simulink library "dummySpool_cl"  (R2020a)
settings: Solver=VariableStepAuto  StartTime=0.0  StopTime=10.0  RelTol=1e-3
undefined symbols (not defined in the file or in its folder): a, courseFollow, courseFollow_cl, desiredMoment, env, exit, FLIGHTCONTROLLER, fltCtrl, freqRollYaw, initializeBussesFromBlock, pathFollowingController, pathFollowingController_cl, rollAmp, rollCtrlKd, rollCtrlKp, rollPhase, rollYawPeriod, takeOffToLandingExp, tsSpool, vhcl, xcurrent, yawAmp, yawCtrlKd, yawCtrlKp, yawPhase
libraries: simulink x4, filteredPIDController_ul x4, angleBtw2Vecs_ul x4, dspsigops x3, pathGeometry_ul x3, ctrlAllocMatrix3Comp_cl x2, setpointToOutput_cl x2, tanFrameProjection_ul x2, vectorNormalizer_ul x2, velocityAngle_ul x2, findClosestPointOnPath_new x1, eulAng2RotMat_ul x1
(part 1 of 2)
settings Model: Creator=jldanie5  LastModifiedBy=andre
settings DataIOCC: ReturnWorkspaceOutputs=off
settings DebuggingCC: ArithmeticOperatorsInVariantConditions=warning
settings SFSimCC: CustomCodeUndefinedFunction=UseInterfaceOnly

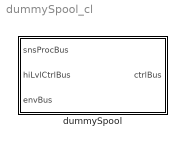
== system dummySpool_cl ==
  dummySpool : Subsystem  LoadFcn=initializeBussesFromBlock(gcb)  InitFcn=initializeBussesFromBlock(gcb)  StartFcn=initializeBussesFromBlock(gcb)  VariantControl=strcmpi(FLIGHTCONTROLLER,'takeoffToLanding')  mask{initPosForInitSStar=vhcl.initPosVecGnd.Value, fluidDensity=env.water.density.Value, pathCtrl=fltCtrl, aeroStruct=vhcl.struct('OCT.aeroSurf')}
      mask prompts: initPosForInitSStar "Initial Position"; fluidDensity "Fluid Density"; pathCtrl "Controller"; aeroStruct "Aerodynamic Structure"
      settings: MinAlgLoopOccurrences=on
      mask DialogControl Container3 Prompt: courseFollow Params
      mask DialogControl Container4 Prompt: setpointToOutput Params

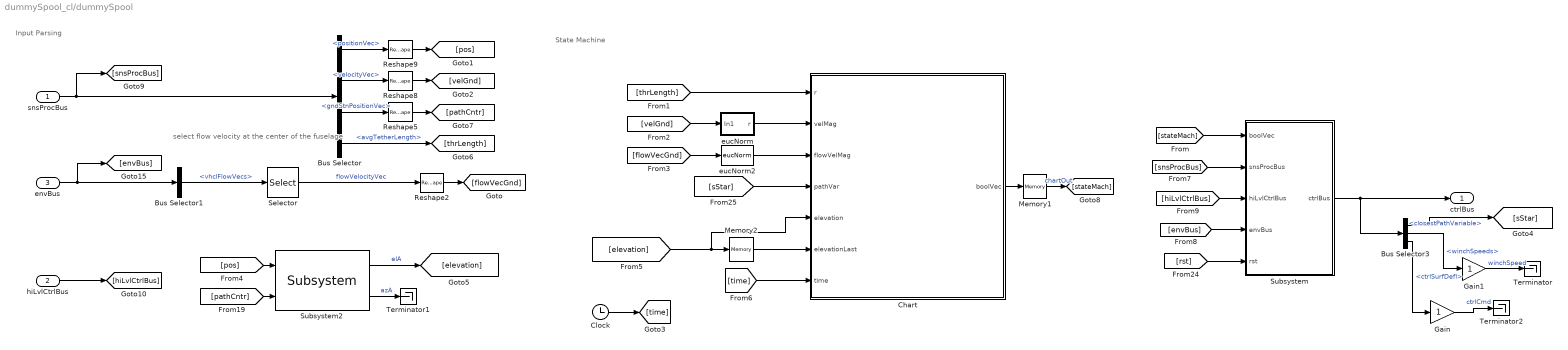
== system dummySpool_cl/dummySpool ==
  note: State Machine
  note: select flow velocity at the center of the fuselage
  note: Input Parsing
  snsProcBus : Inport  OutDataTypeStr=Bus: sensorsProcessingBus
  hiLvlCtrlBus : Inport  Port=2  OutDataTypeStr=Bus: hiLvlCtrlBus
  envBus : Inport  Port=3  OutDataTypeStr=Bus: envBus
  Bus Selector : BusSelector  OutputSignals=positionVec,velocityVec,gndStnPositionVec,avgTetherLength
  Bus Selector1 : BusSelector  OutputSignals=vhclFlowVecs
  Bus Selector3 : BusSelector  OutputSignals=closestPathVariable,winchSpeeds,ctrlSurfDefl
  Chart : Stateflow chart  TreatAsAtomicUnit=on  mask{gain41=fltCtrl.gain4to1.Value, gain23=fltCtrl.gain2to3.Value, maxR=fltCtrl.maxTL.Value, minTL=fltCtrl.initTL.Value, elvPeak=fltCtrl.elvPeak.Value}
      mask prompts: maxR "max kite position magnitude (r)"; minTL "minimum tether length"; elvPeak "elvation peak for phase 1"
  Clock : Clock
  Gain : Gain
  Gain1 : Gain
  Memory1 : Memory  InitialCondition=[1 0 0 0]
  Memory2 : Memory  InitialCondition=.36
  Reshape{2,5,8..9} (4 alike) : Reshape  OutputDimensionality=Column vector (2-D)
  Selector : Selector  NumberOfDimensions=2  InputPortWidth=3  IndexOptions=Select all,Index vector (dialog)  Indices=[1 3],5  OutputSizes=1,1
  Subsystem : Subsystem
  Subsystem2 : hiToLoElevationControllerExp/hiToLoElevationControllerExp/Subsystem  SystemSampleTime=-1  Latency=0  AutoFrameSizeCalculation=off
  Terminator : Terminator
  Terminator1 : Terminator
  Terminator2 : Terminator
  eucNorm : Subsystem
  eucNorm2 : takeoffToLanding_cl/takeoffToLanding/eucNorm  SystemSampleTime=-1  Latency=0  AutoFrameSizeCalculation=off
  ctrlBus : Outport  OutDataTypeStr=Bus: fltCtrlBus  VectorParamsAs1DForOutWhenUnconnected=off
  wires:
  snsProcBus/1 -> [snsProcBus], Bus Selector/1
  Bus Selector/2 -> Reshape8/1  "<velocityVec>"
  Bus Selector/1 -> Reshape9/1  "<positionVec>"
  Reshape2/1 -> [flowVecGnd]
  Reshape8/1 -> [velGnd]
  Reshape9/1 -> [pos]
  Selector/1 -> Reshape2/1  "flowVelocityVec"
  envBus/1 -> [envBus], Bus Selector1/1
  Bus Selector1/1 -> Selector/1  "<vhclFlowVecs>"
  Chart/1(boolVec) -> Memory1/1
  hiLvlCtrlBus/1 -> [hiLvlCtrlBus]
  [flowVecGnd] -> eucNorm2/1
  eucNorm/1(r) -> Chart/2(velMag)
  eucNorm2/1 -> Chart/3(flowVelMag)
  Memory1/1 -> [stateMach]  "chartOut"
  [elevation] -> Chart/5(elevation), Memory2/1
  Memory2/1 -> Chart/6(elevationLast)
  [time] -> Chart/7(time)
  Subsystem2/1 -> [elevation]  "elA"
  [pos] -> Subsystem2/1
  [pathCntr] -> Subsystem2/2
  Subsystem2/2 -> Terminator1/1  "azA"
  Reshape5/1 -> [pathCntr]
  Bus Selector/3 -> Reshape5/1  "<gndStnPositionVec>"
  [velGnd] -> eucNorm/1(In1)
  Bus Selector3/1 -> [sStar]  "<closestPathVariable>"
  [sStar] -> Chart/4(pathVar)
  Subsystem/1(ctrlBus) -> ctrlBus/1, Bus Selector3/1
  [snsProcBus] -> Subsystem/2(snsProcBus)
  [hiLvlCtrlBus] -> Subsystem/3(hiLvlCtrlBus)
  [envBus] -> Subsystem/4(envBus)
  [rst] -> Subsystem/5("rst ")
  [stateMach] -> Subsystem/1(boolVec)
  Bus Selector3/2 -> Gain1/1  "<winchSpeeds>"
  Clock/1 -> [time]
  Bus Selector3/3 -> Gain/1  "<ctrlSurfDefl>"
  Gain/1 -> Terminator2/1  "ctrlCmd"
  Gain1/1 -> Terminator/1  "winchSpeed"
  Bus Selector/4 -> [thrLength]  "<avgTetherLength>"
  [thrLength] -> Chart/1(r)

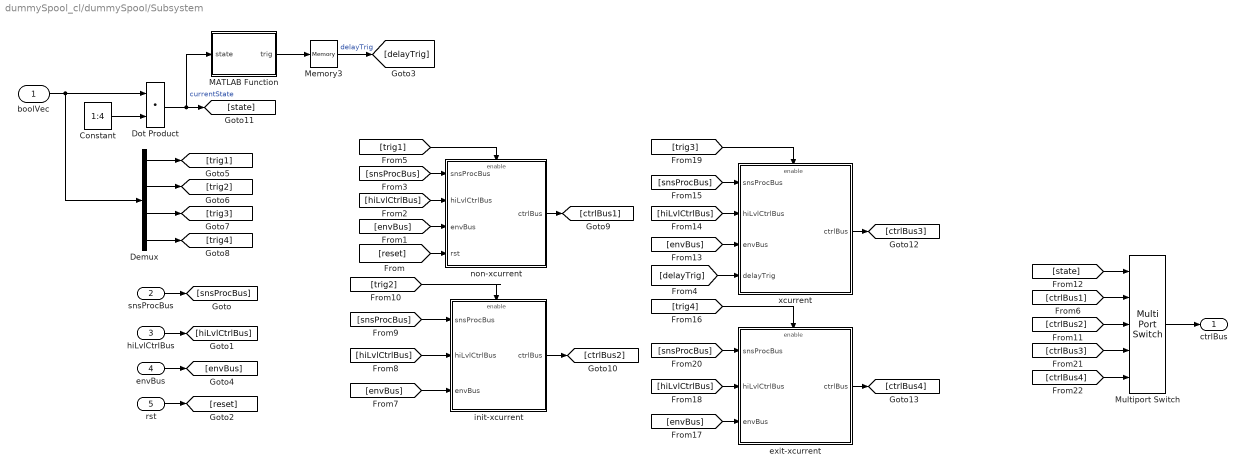
== system dummySpool_cl/dummySpool/Subsystem ==
  boolVec : Inport
  snsProcBus : Inport  Port=2
  hiLvlCtrlBus : Inport  Port=3
  envBus : Inport  Port=4
  "rst " : Inport  Port=5
  Constant : Constant  Value=1:4
  Demux : Demux
  Dot Product : DotProduct  InputSameDT=on  OutDataTypeStr=Inherit: Inherit via internal rule
  MATLAB Function : MATLAB Function  TreatAsAtomicUnit=on
  Memory3 : Memory
  Multiport Switch : MultiPortSwitch  Inputs=4  DataPortIndices={1,2,3,4,5,6}  DiagnosticForDefault=Warning
  exit-xcurrent : Subsystem  TreatAsAtomicUnit=on
  init-xcurrent : Subsystem  TreatAsAtomicUnit=on
  non-xcurrent : Subsystem  TreatAsAtomicUnit=on
  xcurrent : Subsystem  TreatAsAtomicUnit=on
  ctrlBus : Outport
  wires:
  [snsProcBus] -> init-xcurrent/1(snsProcBus)
  boolVec/1 -> Demux/1, Dot Product/1
  [hiLvlCtrlBus] -> init-xcurrent/2(hiLvlCtrlBus)
  Dot Product/1 -> [state], MATLAB Function/1(state)  "currentState"
  [envBus] -> init-xcurrent/3(envBus)
  Constant/1 -> Dot Product/2
  MATLAB Function/1(trig) -> Memory3/1
  Memory3/1 -> [delayTrig]  "delayTrig"
  Multiport Switch/1 -> ctrlBus/1
  [delayTrig] -> xcurrent/4(delayTrig)
  snsProcBus/1 -> [snsProcBus]
  envBus/1 -> [envBus]
  "rst "/1 -> [reset]
  hiLvlCtrlBus/1 -> [hiLvlCtrlBus]
  [reset] -> non-xcurrent/4("rst ")
  [envBus] -> non-xcurrent/3(envBus)
  [hiLvlCtrlBus] -> non-xcurrent/2(hiLvlCtrlBus)
  [snsProcBus] -> non-xcurrent/1(snsProcBus)
  Demux/1 -> [trig1]
  Demux/2 -> [trig2]
  Demux/3 -> [trig3]
  Demux/4 -> [trig4]
  [trig1] -> non-xcurrent/Enable
  non-xcurrent/1(ctrlBus) -> [ctrlBus1]
  [ctrlBus1] -> Multiport Switch/2
  [trig2] -> init-xcurrent/Enable
  init-xcurrent/1(ctrlBus) -> [ctrlBus2]
  [ctrlBus2] -> Multiport Switch/3
  [state] -> Multiport Switch/1
  [snsProcBus] -> xcurrent/1(snsProcBus)
  [hiLvlCtrlBus] -> xcurrent/2(hiLvlCtrlBus)
  [envBus] -> xcurrent/3(envBus)
  [trig3] -> xcurrent/Enable
  [trig4] -> exit-xcurrent/Enable
  [snsProcBus] -> exit-xcurrent/1(snsProcBus)
  [hiLvlCtrlBus] -> exit-xcurrent/2(hiLvlCtrlBus)
  [envBus] -> exit-xcurrent/3(envBus)
  xcurrent/1(ctrlBus) -> [ctrlBus3]
  exit-xcurrent/1(ctrlBus) -> [ctrlBus4]
  [ctrlBus3] -> Multiport Switch/4
  [ctrlBus4] -> Multiport Switch/5

== system dummySpool_cl/dummySpool/eucNorm ==
  In1 : Inport
  Dot Product1 : DotProduct  InputSameDT=on  OutDataTypeStr=Inherit: Inherit via internal rule
  Reshape1 : Reshape
  Sqrt : Sqrt  SaturateOnIntegerOverflow=on
  r : Outport
  wires:
  Sqrt/1 -> Reshape1/1
  In1/1 -> Dot Product1/2, Dot Product1/1
  Reshape1/1 -> r/1  "r"
  Dot Product1/1 -> Sqrt/1

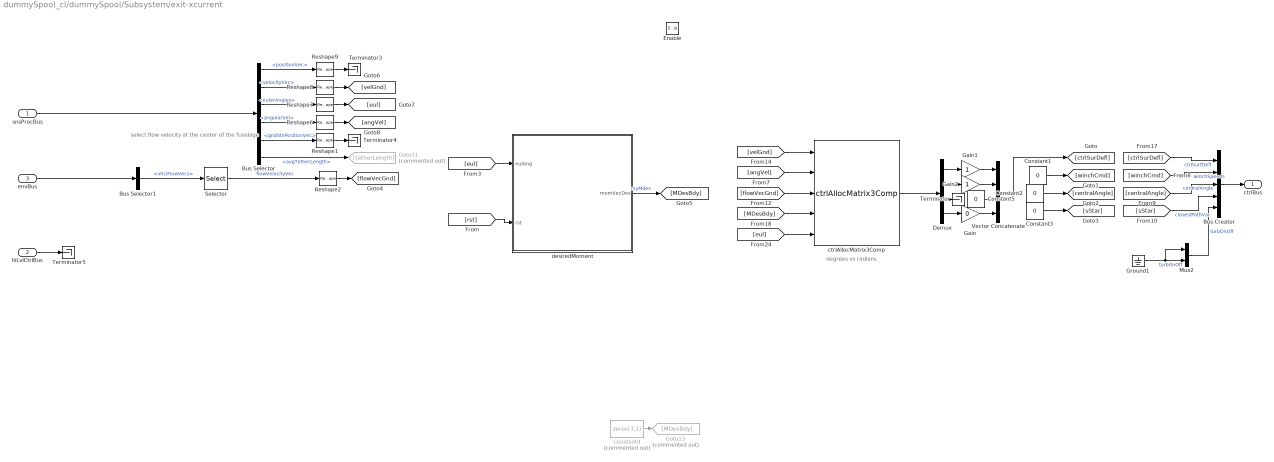
== system dummySpool_cl/dummySpool/Subsystem/exit-xcurrent ==
  note: degrees vs radians
  note: select flow velocity at the center of the fuselage
  snsProcBus : Inport  OutDataTypeStr=Bus: sensorsProcessingBus
  hiLvlCtrlBus : Inport  Port=2  OutDataTypeStr=Bus: hiLvlCtrlBus
  envBus : Inport  Port=3  OutDataTypeStr=Bus: envBus
  Enable : EnablePort
  Bus Creator : BusCreator  Inputs=5  OutDataTypeStr=Bus: fltCtrlBus
      settings: InheritFromInputs=off
  Bus Selector : BusSelector  OutputSignals=positionVec,velocityVec,eulerAngles,angularVel,gndStnPositionVec,avgTetherLength
  Bus Selector1 : BusSelector  OutputSignals=vhclFlowVecs
  Constant{1..3,5} (4 alike) : Constant  Value=0
  Constant4 : Constant  Commented=on  Value=zeros(3,1)
  Demux : Demux
  Gain : Gain  Gain=0
  Gain1 : Gain
  Gain2 : Gain
  Goto11 : Goto  Commented=on  GotoTag=tetherLength
  Goto13 : Goto  Commented=on  GotoTag=MDesBdy
  Ground1 : Ground
  Mux2 : Mux  Inputs=2
  Reshape{1..2,6..9} (6 alike) : Reshape  OutputDimensionality=Column vector (2-D)
  Selector : Selector  NumberOfDimensions=2  InputPortWidth=3  IndexOptions=Select all,Index vector (dialog)  Indices=[1 3],5  OutputSizes=1,1
  Terminator{,3..5} (4 alike) : Terminator
  Vector Concatenate : Concatenate  NumInputs=4
  ctrlAllocMatrix3Comp : ctrlAllocMatrix3Comp_cl/ctrlAllocMatrix3Comp  aeroStruct=vhcl.struct('OCT.aeroSurf')  fluidDensity=fluidDensity  arms=vhcl.struct('OCT.thrAttch')
  desiredMoment : Subsystem  AncestorBlock=takeOffToLandingExp/takeOffToLandingExp/exit-xcurrent/desiredMoment
  ctrlBus : Outport  OutDataTypeStr=Bus: fltCtrlBus  VectorParamsAs1DForOutWhenUnconnected=off
  wires:
  [sStar] -> Bus Creator/4  "closestPathVar"
  [ctrlSurDefl] -> Bus Creator/1  "ctrlSurfDefl"
  [winchCmd] -> Bus Creator/2  "winchSpeeds"
  Bus Creator/1 -> ctrlBus/1
  [centralAngle] -> Bus Creator/3  "centralAngle"
  Constant1/1 -> [winchCmd]
  Constant2/1 -> [centralAngle]
  Constant3/1 -> [sStar]
  Bus Selector/1 -> Reshape9/1  "<positionVec>"
  Bus Selector/3 -> Reshape7/1  "<eulerAngles>"
  Bus Selector/2 -> Reshape8/1  "<velocityVec>"
  Reshape7/1 -> [eul]
  Bus Selector/4 -> Reshape6/1  "<angularVel>"
  Reshape8/1 -> [velGnd]
  Selector/1 -> Reshape2/1  "flowVelocityVec"
  Reshape9/1 -> Terminator3/1
  Bus Selector/5 -> Reshape1/1  "<gndStnPositionVec>"
  Reshape2/1 -> [flowVecGnd]
  Bus Selector1/1 -> Selector/1  "<vhclFlowVecs>"
  envBus/1 -> Bus Selector1/1
  Reshape1/1 -> Terminator4/1
  snsProcBus/1 -> Bus Selector/1
  Reshape6/1 -> [angVel]
  [flowVecGnd] -> ctrlAllocMatrix3Comp/3
  [angVel] -> ctrlAllocMatrix3Comp/2
  [eul] -> ctrlAllocMatrix3Comp/5
  [MDesBdy] -> ctrlAllocMatrix3Comp/4
  [velGnd] -> ctrlAllocMatrix3Comp/1
  Bus Selector/6 -> Goto11/1  "<avgTetherLength>"
  ctrlAllocMatrix3Comp/1 -> Demux/1
  Vector Concatenate/1 -> [ctrlSurDefl]
  Demux/1 -> Gain1/1
  Demux/2 -> Gain2/1
  Demux/4 -> Gain/1
  Constant4/1 -> Goto13/1
  hiLvlCtrlBus/1 -> Terminator5/1
  Constant5/1 -> Vector Concatenate/3
  Demux/3 -> Terminator/1
  desiredMoment/1(momVecDes) -> [MDesBdy]  "myMdes"
  [eul] -> desiredMoment/1(eulAng)
  [rst] -> desiredMoment/2(rst)
  Gain/1 -> Vector Concatenate/4
  Gain1/1 -> Vector Concatenate/1
  Gain2/1 -> Vector Concatenate/2
  Mux2/1 -> Bus Creator/5  "turbOnOff"
  Ground1/1 -> Mux2/2, Mux2/1  "turbOnOff"

== system dummySpool_cl/dummySpool/Subsystem/init-xcurrent ==
  snsProcBus : Inport  OutDataTypeStr=Bus: sensorsProcessingBus
  hiLvlCtrlBus : Inport  Port=2  OutDataTypeStr=Bus: hiLvlCtrlBus
  envBus : Inport  Port=3  OutDataTypeStr=Bus: envBus
  Enable : EnablePort
  Bus Creator : BusCreator  Inputs=5  OutDataTypeStr=Bus: fltCtrlBus
      settings: InheritFromInputs=off
  Constant : Constant  Value=[0 0 fltCtrl.phase2Elevator.Value 0]'
  Constant1 : Constant  Value=0
  Constant2 : Constant  Value=0
  Constant3 : Constant  Value=0
  Ground{,1..3} (4 alike) : Ground
  Mux2 : Mux  Inputs=2
  Terminator : Terminator
  Terminator1 : Terminator
  Terminator2 : Terminator
  ctrlBus : Outport  OutDataTypeStr=Bus: fltCtrlBus  VectorParamsAs1DForOutWhenUnconnected=off
  wires:
  [ctrlSurDefl] -> Bus Creator/1  "ctrlSurfDefl"
  Ground1/1 -> Bus Creator/3  "centralAngle"
  Ground/1 -> Bus Creator/2  "winchSpeeds"
  envBus/1 -> Terminator1/1
  hiLvlCtrlBus/1 -> Terminator2/1
  Constant2/1 -> [centralAngle]
  snsProcBus/1 -> Terminator/1
  Ground2/1 -> Bus Creator/4  "closestPathVariable"
  Constant1/1 -> [winchCmd]
  Bus Creator/1 -> ctrlBus/1
  Constant3/1 -> [sStar]
  Constant/1 -> [ctrlSurDefl]
  Ground3/1 -> Mux2/2, Mux2/1  "turbOnOff"
  Mux2/1 -> Bus Creator/5  "turbOnOff"

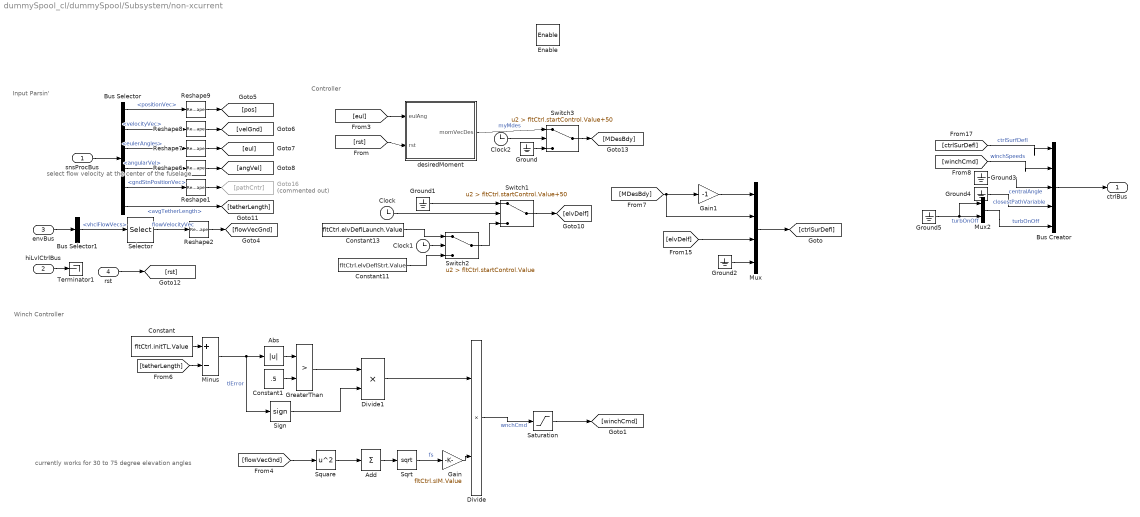
== system dummySpool_cl/dummySpool/Subsystem/non-xcurrent ==
  note: Controller
  note: Input Parsin'
  note: Winch Controller
  note: select flow velocity at the center of the fuselage
  note: currently works for 30 to 75 degree elevation angles
  snsProcBus : Inport  OutDataTypeStr=Bus: sensorsProcessingBus
  hiLvlCtrlBus : Inport  Port=2  OutDataTypeStr=Bus: hiLvlCtrlBus
  envBus : Inport  Port=3  OutDataTypeStr=Bus: envBus
  "rst " : Inport  Port=4
  Enable : EnablePort
  Abs : Abs
  Add : Sum  Inputs=+
  Bus Creator : BusCreator  Inputs=5  OutDataTypeStr=Bus: fltCtrlBus
      settings: InheritFromInputs=off
  Bus Selector : BusSelector  OutputSignals=positionVec,velocityVec,eulerAngles,angularVel,gndStnPositionVec,avgTetherLength
  Bus Selector1 : BusSelector  OutputSignals=vhclFlowVecs
  Clock : Clock
  Clock1 : Clock
  Clock2 : Clock
  Constant : Constant  Value=fltCtrl.initTL.Value
  Constant1 : Constant  Value=.5
  Constant11 : Constant  Value=fltCtrl.elvDeflStrt.Value
  Constant13 : Constant  Value=fltCtrl.elvDeflLaunch.Value
  Divide : Product  Inputs=**
  Divide1 : Product  Inputs=**
  Gain : Gain  Gain=fltCtrl.sIM.Value
  Gain1 : Gain  Gain=-1
  Goto16 : Goto  Commented=on  GotoTag=pathCntr
  GreaterThan : RelationalOperator  Operator=>  OutDataTypeStr=boolean  RndMeth=Simplest
  Ground{,1..5} (6 alike) : Ground
  Minus : Sum  Inputs=+-
  Mux : Mux
  Mux2 : Mux  Inputs=2
  Reshape{1..2,6..9} (6 alike) : Reshape  OutputDimensionality=Column vector (2-D)
  Saturation : Saturate  UpperLimit=0  LowerLimit=-inf
  Selector : Selector  NumberOfDimensions=2  InputPortWidth=3  IndexOptions=Select all,Index vector (dialog)  Indices=[1 3],5  OutputSizes=1,1
  Sign : Signum
  Sqrt : Sqrt  SaturateOnIntegerOverflow=on
  Square : Math  Operator=square  SignedPower=on  SaturateOnIntegerOverflow=on
  Switch1 : Switch  Criteria=u2 > Threshold  Threshold=fltCtrl.startControl.Value+50
  Switch2 : Switch  Criteria=u2 > Threshold  Threshold=fltCtrl.startControl.Value
  Switch3 : Switch  Criteria=u2 > Threshold  Threshold=fltCtrl.startControl.Value+50
  Terminator1 : Terminator
  desiredMoment : Subsystem
  ctrlBus : Outport  OutDataTypeStr=Bus: fltCtrlBus  VectorParamsAs1DForOutWhenUnconnected=off
  wires:
  Ground4/1 -> Bus Creator/4  "closestPathVariable"
  [ctrlSurDefl] -> Bus Creator/1  "ctrlSurfDefl"
  [winchCmd] -> Bus Creator/2  "winchSpeeds"
  Bus Creator/1 -> ctrlBus/1
  Ground3/1 -> Bus Creator/3  "centralAngle"
  desiredMoment/1(momVecDes) -> Switch3/1  "myMdes"
  Bus Selector/1 -> Reshape9/1  "<positionVec>"
  Bus Selector/3 -> Reshape7/1  "<eulerAngles>"
  Bus Selector/2 -> Reshape8/1  "<velocityVec>"
  Reshape7/1 -> [eul]
  Bus Selector/4 -> Reshape6/1  "<angularVel>"
  Reshape8/1 -> [velGnd]
  Selector/1 -> Reshape2/1  "flowVelocityVec"
  Reshape9/1 -> [pos]
  Bus Selector/5 -> Reshape1/1  "<gndStnPositionVec>"
  Reshape2/1 -> [flowVecGnd]
  Bus Selector1/1 -> Selector/1  "<vhclFlowVecs>"
  envBus/1 -> Bus Selector1/1
  Reshape1/1 -> Goto16/1
  snsProcBus/1 -> Bus Selector/1
  Reshape6/1 -> [angVel]
  [eul] -> desiredMoment/1(eulAng)
  [flowVecGnd] -> Square/1
  Add/1 -> Sqrt/1
  Bus Selector/6 -> [tetherLength]  "<avgTetherLength>"
  Constant/1 -> Minus/1
  Minus/1 -> Sign/1, Abs/1  "tlError"
  [tetherLength] -> Minus/2
  Sqrt/1 -> Gain/1  "fs"
  Square/1 -> Add/1
  "rst "/1 -> [rst]
  hiLvlCtrlBus/1 -> Terminator1/1
  [rst] -> desiredMoment/2(rst)
  Mux/1 -> [ctrlSurDefl]
  Abs/1 -> GreaterThan/1
  Constant1/1 -> GreaterThan/2
  Gain/1 -> Divide/2
  Divide/1 -> Saturation/1  "wnchCmd"
  Sign/1 -> Divide1/2
  Divide1/1 -> Divide/1
  GreaterThan/1 -> Divide1/1
  Saturation/1 -> [winchCmd]
  [elvDelf] -> Mux/3
  Constant11/1 -> Switch2/3
  Clock/1 -> Switch1/2
  Ground2/1 -> Mux/4
  Switch1/1 -> [elvDelf]
  Switch2/1 -> Switch1/3
  Clock1/1 -> Switch2/2
  Constant13/1 -> Switch2/1
  Switch3/1 -> [MDesBdy]
  Clock2/1 -> Switch3/2
  Gain1/1 -> Mux/1
  [MDesBdy] -> Mux/2, Gain1/1
  Ground/1 -> Switch3/3
  Ground1/1 -> Switch1/1
  Mux2/1 -> Bus Creator/5  "turbOnOff"
  Ground5/1 -> Mux2/2, Mux2/1  "turbOnOff"

== system dummySpool_cl/dummySpool/Subsystem/xcurrent ==
  snsProcBus : Inport  OutDataTypeStr=Bus: sensorsProcessingBus
  hiLvlCtrlBus : Inport  Port=2  OutDataTypeStr=Bus: hiLvlCtrlBus
  envBus : Inport  Port=3  OutDataTypeStr=Bus: envBus
  delayTrig : Inport  Port=4
  Enable : EnablePort
  Constant : Constant  Value=fltCtrl.controllerEnable.Value
  Switch : Switch  Criteria=u2 > Threshold
  pathFollowingController : Subsystem  Commented=on  AncestorBlock=pathFollowingController_cl/pathFollowingController  LoadFcn=initializeBussesFromBlock(gcb)  InitFcn=initializeBussesFromBlock(gcb)  StartFcn=initializeBussesFromBlock(gcb)  VariantControl=strcmpi(FLIGHTCONTROLLER,'pathFollowingController')  mask{initPosForInitSStar=vhcl.initPosVecGnd.Value, fluidDensity=env.water.density.Value, pathCtrl=fltCtrl, aeroStruct=vhcl.struct('OCT.aeroSurf')}
      mask prompts: initPosForInitSStar "Initial Position"; fluidDensity "Fluid Density"; pathCtrl "Controller"; aeroStruct "Aerodynamic Structure"
      settings: MinAlgLoopOccurrences=on
      mask DialogControl Container3 Prompt: courseFollow Params
      mask DialogControl Container4 Prompt: setpointToOutput Params
  pathFollowingControllerExpStateMachine : pathFollowingControllerExpStateMachine_cl/pathFollowingControllerExpStateMachine  VariantControl=strcmpi(FLIGHTCONTROLLER,'pathFollowingControllerMantaBandLin')  initPosForInitSStar=vhcl.initPosVecGnd.Value  fluidDensity=env.water.density.Value  pathCtrl=fltCtrl  aeroStruct=vhcl.struct('OCT.aeroSurf')  thrAttach=vhcl.rBridle_LE.Value  vhcl=vhcl
  periodicCtrlExpStateMachine : periodicCtrlExpStateMachine/periodicCtrlExpStateMachine  fltCtrl=fltCtrl
  ctrlBus : Outport  OutDataTypeStr=Bus: fltCtrlBus  VectorParamsAs1DForOutWhenUnconnected=off
  wires:
  delayTrig/1 -> [delayTrig]
  [snsProcBus] -> pathFollowingControllerExpStateMachine/1
  [hiLvlCtrlBus] -> pathFollowingControllerExpStateMachine/2
  [envBus] -> pathFollowingControllerExpStateMachine/3
  envBus/1 -> [envBus]
  hiLvlCtrlBus/1 -> [hiLvlCtrlBus]
  snsProcBus/1 -> [snsProcBus]
  [envBus] -> periodicCtrlExpStateMachine/3
  [hiLvlCtrlBus] -> periodicCtrlExpStateMachine/2
  [snsProcBus] -> periodicCtrlExpStateMachine/1
  Switch/1 -> ctrlBus/1
  pathFollowingControllerExpStateMachine/1 -> Switch/1
  periodicCtrlExpStateMachine/1 -> Switch/3
  Constant/1 -> Switch/2
  [delayTrig] -> periodicCtrlExpStateMachine/4
  [delayTrig] -> pathFollowingControllerExpStateMachine/4

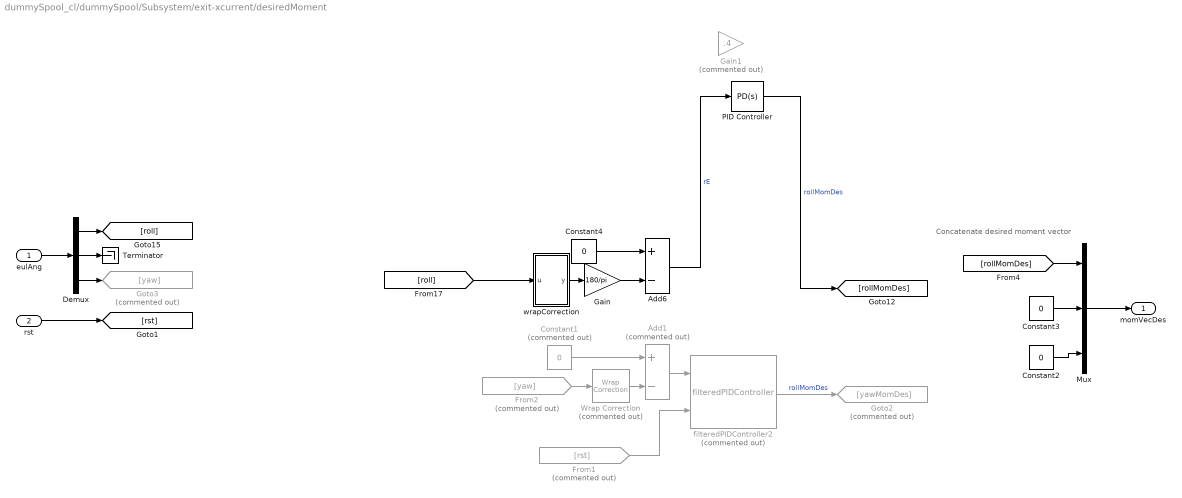
== system dummySpool_cl/dummySpool/Subsystem/exit-xcurrent/desiredMoment ==
  note: Concatenate desired moment vector
  eulAng : Inport
  rst : Inport  Port=2
  Add1 : Sum  Commented=on  Inputs=+-
  Add6 : Sum  Inputs=+-
  Constant1 : Constant  Commented=on  Value=0
  Constant2 : Constant  Value=0
  Constant3 : Constant  Value=0
  Constant4 : Constant  Value=0
  Demux : Demux  Outputs=3
  From1 : From  Commented=on  GotoTag=rst
  From2 : From  Commented=on  GotoTag=yaw
  Gain : Gain  Gain=180/pi
  Gain1 : Gain  Commented=on  Gain=.4
  Goto2 : Goto  Commented=on  GotoTag=yawMomDes
  Goto3 : Goto  Commented=on  GotoTag=yaw
  Mux : Mux  Inputs=3
  PID Controller : simulink/Continuous/PID Controller  Controller=PD  Form=Parallel  TimeDomain=Continuous-time  UseExternalTs=off  SampleTime=-1  IntegratorMethod=Forward Euler  FilterMethod=Forward Euler  ControllerParametersSource=internal  P=fltCtrl.rollMomentPhase1.kp.Value  I=1  D=fltCtrl.rollMomentPhase1.kd.Value  UseFilter=on  N=fltCtrl.rollMomentPhase1.tau.Value  TunerSelectOption=Transfer Function Based (PID Tuner App)  InitialConditionSource=internal  InitialConditionForIntegrator=0  InitialConditionForFilter=0  DifferentiatorICPrevScaledInput=0  ExternalReset=none  TrackingMode=off  Kt=1  LimitOutput=off  UpperSaturationLimit=inf  LowerSaturationLimit=-inf  LinearizeAsGain=on  AntiWindupMode=none  Kb=1  POutMin=[]  POutMax=[]  IOutMin=[]  IOutMax=[]  DOutMin=[]  DOutMax=[]  NOutMin=[]  NOutMax=[]  SumOutMin=[]  SumOutMax=[]  SaturationOutMin=[]  SaturationOutMax=[]  PParamMin=[]  PParamMax=[]  IParamMin=[]  IParamMax=[]  DParamMin=[]  DParamMax=[]  NParamMin=[]  NParamMax=[]  KbParamMin=[]  KbParamMax=[]  KtParamMin=[]  KtParamMax=[]  KbOutMin=[]  KbOutMax=[]  KtOutMin=[]  KtOutMax=[]  IntegratorOutMin=[]  IntegratorOutMax=[]  FilterOutMin=[]  FilterOutMax=[]  SumI1OutMin=[]  SumI1OutMax=[]  SumI2OutMin=[]  SumI2OutMax=[]  SumI3OutMin=[]  SumI3OutMax=[]  SumI4OutMin=[]  SumI4OutMax=[]  SumDOutMin=[]  SumDOutMax=[]  DifferentiatorOutMin=[]  DifferentiatorOutMax=[]  FilterDiffOutCoefMin=[]  FilterDiffOutCoefMax=[]  ReciprocalOutMin=[]  ReciprocalOutMax=[]  SumDenOutMin=[]  SumDenOutMax=[]  SumNumOutMin=[]  SumNumOutMax=[]  DivideOutMin=[]  DivideOutMax=[]  UdiffTsProdOutMin=[]  UdiffTsProdOutMax=[]  NTsProdOutMin=[]  NTsProdOutMax=[]  UintegralTsProdOutMin=[]  UintegralTsProdOutMax=[]  UngainTsProdOutMin=[]  UngainTsProdOutMax=[]  IntegratorContinuousStateAttributes=''  IntegratorStateMustResolveToSignalObject=off  IntegratorRTWStateStorageClass=Auto  FilterContinuousStateAttributes=''  FilterStateMustResolveToSignalObject=off  FilterRTWStateStorageClass=Auto  ParallelPVariant=InternalParameters  IdealPVariant=Disabled  IVariant=Disabled  DVariant=InternalParameters  IntegratorVariant=Disabled  SatVariant=Disabled  AWVariant=Disabled  PCopyVariant=Disabled  TRVariant=Disabled  FdbkBlocksVariant=Forward  IdealPFdbkVariant=Disabled  SatFdbkVariant=Disabled  DerivativeFilterVariant=ContFilter  NVariant=InternalParameters  NCopyVariant=Disabled  FilterICVariant=InternalICsFilter  IntegratorICVariant=Disabled  ExternalResetVariant=Disabled  TRSumVariant=Passthrough  SumFdbkVariant=Disabled  SumVariant=Sum_PD  TsampFilterVariant=InternalTs  TsampNgainVariant=Passthrough  TsampIntegralVariant=Disabled_SignalSpec
  Terminator : Terminator
  Wrap Correction : setpointToOutput_cl/desiredMoment/Wrap Correction  Commented=on  SystemSampleTime=-1  Latency=0  AutoFrameSizeCalculation=off
  filteredPIDController2 : filteredPIDController_ul/filteredPIDController  Commented=on  kp=pathCtrl.yawMoment.kp.Value  ki=0  kd=pathCtrl.yawMoment.kd.Value  Value=pathCtrl.yawMoment.tau.Value  externalReset=rising
  wrapCorrection : Subsystem
  momVecDes : Outport  VectorParamsAs1DForOutWhenUnconnected=off
  wires:
  Wrap Correction/1 -> Add1/2
  From2/1 -> Wrap Correction/1
  Constant1/1 -> Add1/1
  filteredPIDController2/1 -> Goto2/1  "rollMomDes"
  Add1/1 -> filteredPIDController2/1
  From1/1 -> filteredPIDController2/2
  rst/1 -> [rst]
  Demux/3 -> Goto3/1
  Demux/2 -> Terminator/1
  Constant4/1 -> Add6/1
  Add6/1 -> PID Controller/1  "rE"
  PID Controller/1 -> [rollMomDes]  "rollMomDes"
  eulAng/1 -> Demux/1
  Demux/1 -> [roll]
  Mux/1 -> momVecDes/1
  Constant3/1 -> Mux/2
  [rollMomDes] -> Mux/1
  Constant2/1 -> Mux/3
  Gain/1 -> Add6/2
  [roll] -> wrapCorrection/1(u)
  wrapCorrection/1(y) -> Gain/1

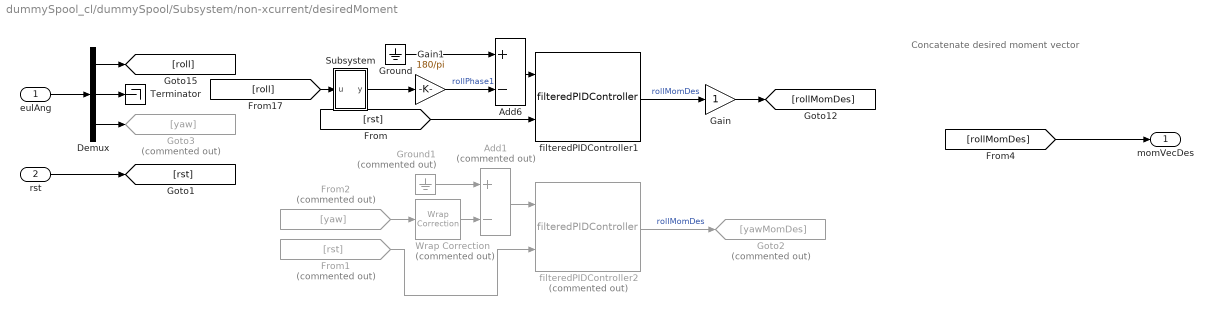
== system dummySpool_cl/dummySpool/Subsystem/non-xcurrent/desiredMoment ==
  note: Concatenate desired moment vector
  eulAng : Inport
  rst : Inport  Port=2
  Add1 : Sum  Commented=on  Inputs=+-
  Add6 : Sum  Inputs=+-
  Demux : Demux  Outputs=3
  From1 : From  Commented=on  GotoTag=rst
  From2 : From  Commented=on  GotoTag=yaw
  Gain : Gain
  Gain1 : Gain  Gain=180/pi
  Goto2 : Goto  Commented=on  GotoTag=yawMomDes
  Goto3 : Goto  Commented=on  GotoTag=yaw
  Ground : Ground
  Ground1 : Ground  Commented=on
  Subsystem : Subsystem
  Terminator : Terminator
  Wrap Correction : setpointToOutput_cl/desiredMoment/Wrap Correction  Commented=on  SystemSampleTime=-1  Latency=0  AutoFrameSizeCalculation=off
  filteredPIDController1 : filteredPIDController_ul/filteredPIDController  kp=fltCtrl.rollMomentPhase1.kp.Value  ki=0  kd=fltCtrl.rollMomentPhase1.kd.Value  Value=fltCtrl.rollMomentPhase1.tau.Value  externalReset=rising
  filteredPIDController2 : filteredPIDController_ul/filteredPIDController  Commented=on  kp=pathCtrl.yawMoment.kp.Value  ki=0  kd=pathCtrl.yawMoment.kd.Value  Value=pathCtrl.yawMoment.tau.Value  externalReset=rising
  momVecDes : Outport  VectorParamsAs1DForOutWhenUnconnected=off
  wires:
  Demux/1 -> [roll]
  eulAng/1 -> Demux/1
  filteredPIDController1/1 -> Gain/1  "rollMomDes"
  Add6/1 -> filteredPIDController1/1
  Demux/2 -> Terminator/1
  Demux/3 -> Goto3/1
  rst/1 -> [rst]
  [rst] -> filteredPIDController1/2
  From1/1 -> filteredPIDController2/2
  Add1/1 -> filteredPIDController2/1
  filteredPIDController2/1 -> Goto2/1  "rollMomDes"
  From2/1 -> Wrap Correction/1
  Wrap Correction/1 -> Add1/2
  Gain/1 -> [rollMomDes]
  Gain1/1 -> Add6/2  "rollPhase1"
  [rollMomDes] -> momVecDes/1
  Ground/1 -> Add6/1
  Ground1/1 -> Add1/1
  [roll] -> Subsystem/1(u)
  Subsystem/1(y) -> Gain1/1

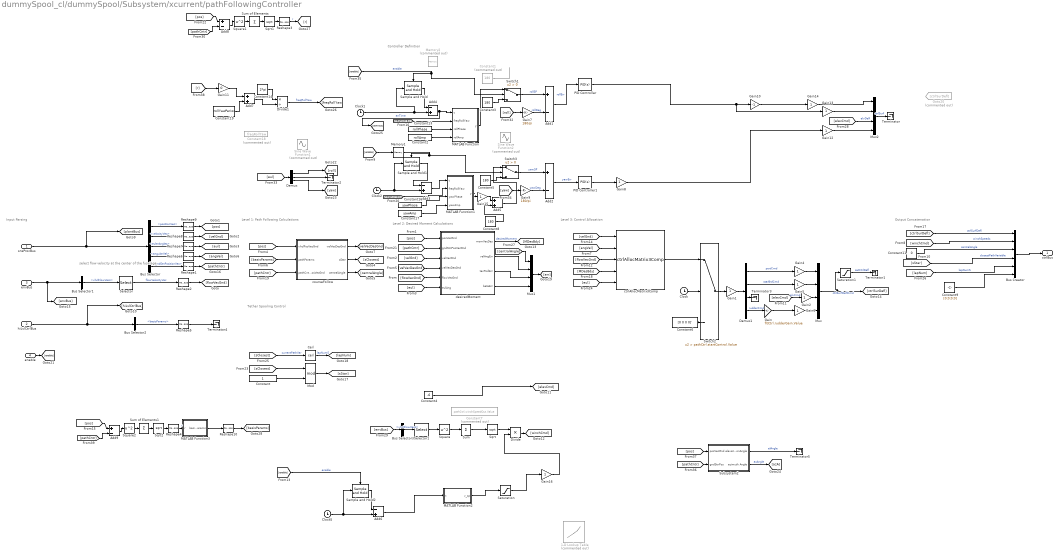
== system dummySpool_cl/dummySpool/Subsystem/xcurrent/pathFollowingController ==
  note: Input Parsing
  note: Level 1: Path Following Calculations
  note: Level 2: Desired Moment Calculations
  note: Tether Spooling Control
  note: Output Concatenation
  note: Level 3: Control Allocation
  note: select flow velocity at the center of the fuselage
  note: Controller Definition
  snsProcBus : Inport  OutDataTypeStr=Bus: sensorsProcessingBus
  hiLvlCtrlBus : Inport  Port=2  OutDataTypeStr=Bus: hiLvlCtrlBus
  envBus : Inport  Port=3  OutDataTypeStr=Bus: envBus
  enable : Inport  Port=4
  1-D Lookup Table : Lookup_n-D  Commented=on  NumberOfTableDimensions=1  BreakpointsForDimension1=tsSpool.Time  Table=tsSpool.Data  ExtrapMethod=Clip  InternalRulePriority=Speed  RndMeth=Simplest  InputSameDT=on
  Add{1..2,8..9} (4 alike) : Sum  Inputs=+-
  Add3 : Sum  Inputs=-+
  Add4 : Sum  Inputs=-+
  Add5 : Sum
  Add6 : Sum  Inputs=-+
  Add7 : Sum
  Bus Creator : BusCreator  Inputs=6  OutDataTypeStr=Bus: fltCtrlBus
      settings: InheritFromInputs=off
  Bus Selector : BusSelector  OutputSignals=positionVec,velocityVec,eulerAngles,angularVel,gndStnPositionVec
  Bus Selector1 : BusSelector  OutputSignals=vhclFlowVecs
  Bus Selector2 : BusSelector  OutputSignals=basisParams
  Bus Selector3 : BusSelector  OutputSignals=vhclFlowVecs
  Ceil : Rounding  Operator=ceil
  Clock{,1..2,5} (4 alike) : Clock
  Constant : Constant
  Constant1 : Constant  Commented=on  Value=180
  Constant11 : Constant  Value=0
  Constant13 : Constant  Value=rollPhase
  Constant14 : Constant  Value=2*pi
  Constant16 : Constant  Value=yawPhase
  Constant17 : Constant  Value=yawAmp
  Constant18 : Constant  Commented=on  Value=freqRollYaw
  Constant19 : Constant  Value=rollYawPeriod
  Constant2 : Constant  Value=rollAmp
  Constant3 : Constant  Value=180
  Constant4 : Constant  Value=-6
  Constant5 : Constant  Value=180
  Constant6 : Constant  Value=[0 0 0 0]'
  Constant7 : Constant  Commented=on  Value=pathCtrl.winchSpeedOut.Value
  Constant8 : Constant  Value=180
  Constant9 : Constant  Value=[0;0;0;0]
  Demux : Demux  Outputs=3
  Demux1 : Demux
  Divide : Product  Inputs=**
  Divide1 : Product  Inputs=*/
  Gain : Gain  Gain=fltCtrl.rudderGain.Value
  Gain{1..2,4..6,8,12..16} (11 alike) : Gain
  Gain10 : Gain  Gain=-1
  Gain11 : Gain  Gain=0
  Gain7 : Gain  Gain=180/pi
  Gain9 : Gain  Gain=180/pi
  Goto20 : Goto  Commented=on  GotoTag=ctrlSurDefl
  MATLAB Function : MATLAB Function  TreatAsAtomicUnit=on
  MATLAB Function1 : MATLAB Function  TreatAsAtomicUnit=on
  MATLAB Function2 : MATLAB Function  TreatAsAtomicUnit=on
  MATLAB Function3 : MATLAB Function  TreatAsAtomicUnit=on
  Memory1 : Memory
  Memory2 : Memory  Commented=on
  Mod : Math  Operator=mod  SaturateOnIntegerOverflow=on
  Mux : Mux
  Mux1 : Mux
  Mux2 : Mux
  PID Controller : simulink/Continuous/PID Controller  Controller=PID  Form=Parallel  TimeDomain=Continuous-time  UseExternalTs=off  SampleTime=-1  IntegratorMethod=Forward Euler  FilterMethod=Forward Euler  ControllerParametersSource=internal  P=rollCtrlKp  I=1  D=rollCtrlKd  UseFilter=on  N=100  TunerSelectOption=Transfer Function Based (PID Tuner App)  InitialConditionSource=internal  InitialConditionForIntegrator=0  InitialConditionForFilter=0  DifferentiatorICPrevScaledInput=0  ExternalReset=none  TrackingMode=off  Kt=1  LimitOutput=off  UpperSaturationLimit=inf  LowerSaturationLimit=-inf  LinearizeAsGain=on  AntiWindupMode=none  Kb=1  POutMin=[]  POutMax=[]  IOutMin=[]  IOutMax=[]  DOutMin=[]  DOutMax=[]  NOutMin=[]  NOutMax=[]  SumOutMin=[]  SumOutMax=[]  SaturationOutMin=[]  SaturationOutMax=[]  PParamMin=[]  PParamMax=[]  IParamMin=[]  IParamMax=[]  DParamMin=[]  DParamMax=[]  NParamMin=[]  NParamMax=[]  KbParamMin=[]  KbParamMax=[]  KtParamMin=[]  KtParamMax=[]  KbOutMin=[]  KbOutMax=[]  KtOutMin=[]  KtOutMax=[]  IntegratorOutMin=[]  IntegratorOutMax=[]  FilterOutMin=[]  FilterOutMax=[]  SumI1OutMin=[]  SumI1OutMax=[]  SumI2OutMin=[]  SumI2OutMax=[]  SumI3OutMin=[]  SumI3OutMax=[]  SumI4OutMin=[]  SumI4OutMax=[]  SumDOutMin=[]  SumDOutMax=[]  DifferentiatorOutMin=[]  DifferentiatorOutMax=[]  FilterDiffOutCoefMin=[]  FilterDiffOutCoefMax=[]  ReciprocalOutMin=[]  ReciprocalOutMax=[]  SumDenOutMin=[]  SumDenOutMax=[]  SumNumOutMin=[]  SumNumOutMax=[]  DivideOutMin=[]  DivideOutMax=[]  UdiffTsProdOutMin=[]  UdiffTsProdOutMax=[]  NTsProdOutMin=[]  NTsProdOutMax=[]  UintegralTsProdOutMin=[]  UintegralTsProdOutMax=[]  UngainTsProdOutMin=[]  UngainTsProdOutMax=[]  IntegratorContinuousStateAttributes=''  IntegratorStateMustResolveToSignalObject=off  IntegratorRTWStateStorageClass=Auto  FilterContinuousStateAttributes=''  FilterStateMustResolveToSignalObject=off  FilterRTWStateStorageClass=Auto  ParallelPVariant=InternalParameters  IdealPVariant=Disabled  IVariant=InternalParameters  DVariant=InternalParameters  IntegratorVariant=Continuous  SatVariant=Disabled  AWVariant=Passthrough  PCopyVariant=Disabled  TRVariant=Disabled  FdbkBlocksVariant=Forward  IdealPFdbkVariant=Disabled  SatFdbkVariant=Disabled  DerivativeFilterVariant=ContFilter  NVariant=InternalParameters  NCopyVariant=Disabled  FilterICVariant=InternalICsFilter  IntegratorICVariant=InternalICs  ExternalResetVariant=Disabled  TRSumVariant=Passthrough  SumFdbkVariant=Disabled  SumVariant=Sum_PID  TsampFilterVariant=InternalTs  TsampNgainVariant=Passthrough  TsampIntegralVariant=Passthrough
  PID Controller1 : simulink/Continuous/PID Controller  Controller=PID  Form=Parallel  TimeDomain=Continuous-time  UseExternalTs=off  SampleTime=-1  IntegratorMethod=Forward Euler  FilterMethod=Forward Euler  ControllerParametersSource=internal  P=yawCtrlKp  I=1  D=yawCtrlKd  UseFilter=on  N=100  TunerSelectOption=Transfer Function Based (PID Tuner App)  InitialConditionSource=internal  InitialConditionForIntegrator=0  InitialConditionForFilter=0  DifferentiatorICPrevScaledInput=0  ExternalReset=none  TrackingMode=off  Kt=1  LimitOutput=off  UpperSaturationLimit=inf  LowerSaturationLimit=-inf  LinearizeAsGain=on  AntiWindupMode=none  Kb=1  POutMin=[]  POutMax=[]  IOutMin=[]  IOutMax=[]  DOutMin=[]  DOutMax=[]  NOutMin=[]  NOutMax=[]  SumOutMin=[]  SumOutMax=[]  SaturationOutMin=[]  SaturationOutMax=[]  PParamMin=[]  PParamMax=[]  IParamMin=[]  IParamMax=[]  DParamMin=[]  DParamMax=[]  NParamMin=[]  NParamMax=[]  KbParamMin=[]  KbParamMax=[]  KtParamMin=[]  KtParamMax=[]  KbOutMin=[]  KbOutMax=[]  KtOutMin=[]  KtOutMax=[]  IntegratorOutMin=[]  IntegratorOutMax=[]  FilterOutMin=[]  FilterOutMax=[]  SumI1OutMin=[]  SumI1OutMax=[]  SumI2OutMin=[]  SumI2OutMax=[]  SumI3OutMin=[]  SumI3OutMax=[]  SumI4OutMin=[]  SumI4OutMax=[]  SumDOutMin=[]  SumDOutMax=[]  DifferentiatorOutMin=[]  DifferentiatorOutMax=[]  FilterDiffOutCoefMin=[]  FilterDiffOutCoefMax=[]  ReciprocalOutMin=[]  ReciprocalOutMax=[]  SumDenOutMin=[]  SumDenOutMax=[]  SumNumOutMin=[]  SumNumOutMax=[]  DivideOutMin=[]  DivideOutMax=[]  UdiffTsProdOutMin=[]  UdiffTsProdOutMax=[]  NTsProdOutMin=[]  NTsProdOutMax=[]  UintegralTsProdOutMin=[]  UintegralTsProdOutMax=[]  UngainTsProdOutMin=[]  UngainTsProdOutMax=[]  IntegratorContinuousStateAttributes=''  IntegratorStateMustResolveToSignalObject=off  IntegratorRTWStateStorageClass=Auto  FilterContinuousStateAttributes=''  FilterStateMustResolveToSignalObject=off  FilterRTWStateStorageClass=Auto  ParallelPVariant=InternalParameters  IdealPVariant=Disabled  IVariant=InternalParameters  DVariant=InternalParameters  IntegratorVariant=Continuous  SatVariant=Disabled  AWVariant=Passthrough  PCopyVariant=Disabled  TRVariant=Disabled  FdbkBlocksVariant=Forward  IdealPFdbkVariant=Disabled  SatFdbkVariant=Disabled  DerivativeFilterVariant=ContFilter  NVariant=InternalParameters  NCopyVariant=Disabled  FilterICVariant=InternalICsFilter  IntegratorICVariant=InternalICs  ExternalResetVariant=Disabled  TRSumVariant=Passthrough  SumFdbkVariant=Disabled  SumVariant=Sum_PID  TsampFilterVariant=InternalTs  TsampNgainVariant=Passthrough  TsampIntegralVariant=Passthrough
  Reshape{1..2,5..10} (8 alike) : Reshape  OutputDimensionality=Column vector (2-D)
  Reshape3 : Reshape
  Reshape4 : Reshape
  Sample and Hold : dspsigops/Sample and Hold  trig=Rising edge  initCond=0  latchinput=off
  Sample and Hold1 : dspsigops/Sample and Hold  trig=Rising edge  initCond=0  latchinput=off
  Sample and Hold2 : dspsigops/Sample and Hold  trig=Rising edge  initCond=0  latchinput=off
  Saturation : Saturate  UpperLimit=.125  LowerLimit=0
  Saturation1 : Saturate  UpperLimit=30  LowerLimit=-30
  Selector : Selector  NumberOfDimensions=2  InputPortWidth=3  IndexOptions=Select all,Index vector (dialog)  Indices=[1 3],5  OutputSizes=1,1
  Selector1 : Selector  NumberOfDimensions=2  InputPortWidth=3  IndexOptions=Select all,Index vector (dialog)  Indices=[1 3],5  OutputSizes=1,1
  Sine Wave Function1 : Sin  Commented=on  TimeSource=Use external signal  Amplitude=yawAmp  Frequency=freqRollYaw  Phase=yawPhase  SampleTime=0
  Sine Wave Function2 : Sin  Commented=on  TimeSource=Use external signal  Amplitude=rollAmp  Bias=180  Frequency=freqRollYaw  Phase=rollPhase  SampleTime=0
  Sqrt : Sqrt  SaturateOnIntegerOverflow=on
  Sqrt1 : Sqrt  SaturateOnIntegerOverflow=on
  Sqrt2 : Sqrt  SaturateOnIntegerOverflow=on
  Square : Math  Operator=square  SaturateOnIntegerOverflow=on
  Square1 : Math  Operator=square  SaturateOnIntegerOverflow=on
  Square2 : Math  Operator=square  SaturateOnIntegerOverflow=on
  Subsystem2 : Subsystem  AncestorBlock=hiToLoElevationControllerExp/hiToLoElevationControllerExp/Subsystem
  Sum : Sum  Inputs=+
  Sum of Elements : Sum  Inputs=+
  Sum of Elements1 : Sum  Inputs=+
  Switch1 : Switch  Criteria=u2 > Threshold
  Switch2 : Switch  Criteria=u2 > Threshold  Threshold=pathCtrl.startControl.Value
  Switch3 : Switch  Criteria=u2 > Threshold
  Terminator{,1..5} (6 alike) : Terminator
  courseFollow : Subsystem  AncestorBlock=courseFollow_cl/courseFollow
  ctrlAllocMatrix3Comp : ctrlAllocMatrix3Comp_cl/ctrlAllocMatrix3Comp  aeroStruct=vhcl.struct('OCT.aeroSurf')  fluidDensity=fluidDensity  arms=vhcl.struct('OCT.thrAttch')
  desiredMoment : Subsystem  AncestorBlock=setpointToOutput_cl/desiredMoment
  ctrlBus : Outport  OutDataTypeStr=Bus: fltCtrlBus  VectorParamsAs1DForOutWhenUnconnected=off
  wires:
  Constant9/1 -> Bus Creator/6
  Mux1/1 -> [err]
  [centralAngle] -> Mux1/1
  desiredMoment/2(velAngErr) -> Mux1/2
  desiredMoment/3(tanRollErr) -> Mux1/3
  desiredMoment/4(betaErr) -> Mux1/4
  [lapNum] -> Bus Creator/5  "lapNumS"
  Mod/1 -> [sStar]
  [sClosest] -> Mod/1
  Constant/1 -> Mod/2
  Ceil/1 -> [lapNum]  "lapNumS"
  [sClosest] -> Ceil/1  "currentPathVar"
  Demux1/4 -> Gain/1  "rudderCmd"
  Gain/1 -> Gain6/1
  [basisParams] -> courseFollow/2(pathParams)
  [flowVecGnd] -> desiredMoment/5(flowVecGnd)
  [eul] -> desiredMoment/6(eulAng)
  [velVecDesGnd] -> desiredMoment/4(velVecDesGnd)
  [velGnd] -> desiredMoment/3(velVecGnd)
  [pathCntr] -> desiredMoment/2(gndStnPosVecGnd)
  [pos] -> desiredMoment/1(posVecGnd)
  [pathCntr] -> courseFollow/3(pathCntrPosVecGnd)
  Bus Selector/5 -> Reshape1/1  "<gndStnPositionVec>"
  Reshape1/1 -> [pathCntr]
  Bus Selector1/1 -> Selector/1  "<vhclFlowVecs>"
  envBus/1 -> Bus Selector1/1, [envBus]
  Selector/1 -> Reshape2/1  "flowVelocityVec"
  [eul] -> ctrlAllocMatrix3Comp/5
  Reshape9/1 -> [pos]
  Reshape8/1 -> [velGnd]
  Reshape7/1 -> [eul]
  Reshape6/1 -> [angVel]
  Reshape2/1 -> [flowVecGnd]
  Mux/1 -> Saturation1/1, [ctrlSurDefl]  "ctrlSurfDeflCmd"
  Reshape5/1 -> Terminator4/1
  Bus Selector2/1 -> Reshape5/1  "<basisParams>"
  [ctrlSurDefl] -> Bus Creator/1  "ctrlSurfDefl"
  ctrlAllocMatrix3Comp/1 -> Switch2/1
  [MDesBdy] -> ctrlAllocMatrix3Comp/4
  Constant6/1 -> Switch2/3
  Switch2/1 -> Gain1/1
  Clock/1 -> Switch2/2
  Demux1/2 -> Gain5/1  "starBrdCmd"
  Demux1/1 -> Gain4/1  "portCmd"
  Demux1/3 -> Terminator3/1
  [elevCmd] -> Gain2/1  "elvCmd"
  [flowVecGnd] -> ctrlAllocMatrix3Comp/3
  [velGnd] -> ctrlAllocMatrix3Comp/1
  [angVel] -> ctrlAllocMatrix3Comp/2
  Bus Selector/4 -> Reshape6/1  "<angularVel>"
  desiredMoment/1(momVecDes) -> [MDesBdy]  "desiredMoment"
  courseFollow/3(centralAngle) -> [centralAngle]
  [sStar] -> Bus Creator/4  "closestPathVariable"
  Constant11/1 -> Bus Creator/3  "centralAngle"
  hiLvlCtrlBus/1 -> Bus Selector2/1, [hiLvlCtrlBus]
  courseFollow/2(sStar) -> [sClosest]
  [winchCmd] -> Bus Creator/2  "winchSpeeds"
  Bus Creator/1 -> ctrlBus/1
  [pos] -> courseFollow/1("vhclPosVecGnd ")
  Bus Selector/3 -> Reshape7/1  "<eulerAngles>"
  Bus Selector/1 -> Reshape9/1  "<positionVec>"
  Bus Selector/2 -> Reshape8/1  "<velocityVec>"
  snsProcBus/1 -> Bus Selector/1, [plantBus]
  courseFollow/1(velVecDesGnd) -> [velVecDesGnd]
  Gain1/1 -> Demux1/1
  Gain2/1 -> Mux/3
  [envBus] -> Bus Selector3/1
  Selector1/1 -> Square/1
  Divide/1 -> [winchCmd]
  Bus Selector3/1 -> Selector1/1  "<vhclFlowVecs>"
  Square/1 -> Sum/1
  Sum/1 -> Sqrt/1
  Sqrt/1 -> Divide/1
  Saturation/1 -> Gain16/1
  Constant4/1 -> [elevCmd]
  Gain4/1 -> Mux/1
  Gain5/1 -> Mux/2
  Gain6/1 -> Mux/4
  [enable] -> Memory1/1
  Clock2/1 -> Add3/2, Sample and Hold1/1
  Add1/1 -> PID Controller/1  "rollErr"
  Gain9/1 -> Add2/2  "yawDeg"
  [yaw] -> Gain9/1
  [roll] -> Gain7/1
  MATLAB Function/1(y) -> Switch1/1
  Sample and Hold1/1 -> Add3/1
  Gain7/1 -> Add1/2  "rollDeg"
  [enable] -> Switch1/2, Sample and Hold/Trigger  "enable"
  [elevCmd] -> Mux2/3  "elvDelf"
  Add4/1 -> [enTime], MATLAB Function/1(t)  "enTime"
  Clock1/1 -> Sample and Hold/1, Add4/2
  Constant3/1 -> Switch1/3
  Constant5/1 -> Switch3/3
  Sample and Hold/1 -> Add4/1
  Gain8/1 -> Gain12/1
  Switch1/1 -> Add1/1  "rollSP"
  Constant8/1 -> Add5/2
  Add2/1 -> PID Controller1/1  "yawErr"
  Gain10/1 -> Gain14/1
  Add3/1 -> MATLAB Function1/1(t)
  Switch3/1 -> Add2/1  "yawSP"
  Add5/1 -> Switch3/1
  enable/1 -> [enable]
  PID Controller/1 -> Gain13/1, Gain10/1
  PID Controller1/1 -> Gain8/1
  [eul] -> Demux/1
  Demux/1 -> [roll]
  Demux/3 -> [yaw]
  Demux/2 -> Terminator2/1
  Subsystem2/2(azimuth Angle) -> [azA]  "azAngle"
  Subsystem2/1(elevationAngle) -> Terminator5/1  "elAngle"
  [pos] -> Subsystem2/1(posVecGnd)
  [pathCntr] -> Subsystem2/2(gndStnPos)
  Add6/1 -> MATLAB Function2/1(t)
  Memory1/1 -> Switch3/2, Sample and Hold1/Trigger
  [enable] -> Sample and Hold2/Trigger  "enable"
  Sample and Hold2/1 -> Add6/1
  Clock5/1 -> Sample and Hold2/1, Add6/2
  Constant2/1 -> MATLAB Function/4(rollAmp)
  Constant13/1 -> MATLAB Function/3(rollPhase)
  [freqRollYaw] -> MATLAB Function/2(freqRollYaw)
  MATLAB Function1/1(y) -> Gain15/1
  [freqRollYaw] -> MATLAB Function1/2(freqRollYaw)
  Constant16/1 -> MATLAB Function1/3(yawPhase)
  Constant17/1 -> MATLAB Function1/4(yawAmp)
  Constant19/1 -> Add7/2
  [r] -> Gain11/1
  Gain11/1 -> Add7/1
  Add7/1 -> Divide1/2
  Constant14/1 -> Divide1/1
  Divide1/1 -> [freqRollYaw]  "freqRollYaw"
  [pos] -> Add8/1
  [pathCntr] -> Add8/2
  Add8/1 -> Square1/1
  Square1/1 -> Sum of Elements/1
  Sum of Elements/1 -> Sqrt1/1
  Sqrt1/1 -> Reshape3/1
  Reshape3/1 -> [r]  "r"
  Gain12/1 -> Mux2/4
  Gain13/1 -> Mux2/2
  Gain14/1 -> Mux2/1
  Constant1/1 -> ?
  Gain15/1 -> Add5/1
  Gain16/1 -> Divide/2
  MATLAB Function2/1(v_sp) -> Saturation/1
  Mux2/1 -> Terminator/1  "ctrlSurf"
  Saturation1/1 -> Terminator1/1  "satCtrlDefl"
  [pathCntr] -> Add9/2
  [pos] -> Add9/1
  Square2/1 -> Sum of Elements1/1
  Add9/1 -> Square2/1
  Sqrt2/1 -> Reshape4/1
  Sum of Elements1/1 -> Sqrt2/1
  Reshape4/1 -> MATLAB Function3/1(r)  "r"
  MATLAB Function3/1(basisParams) -> Reshape10/1
  Reshape10/1 -> [basisParams]

== system dummySpool_cl/dummySpool/Subsystem/exit-xcurrent/desiredMoment/wrapCorrection ==
  u : Inport
  Add2 : Sum  Inputs=+-
  Add3 : Sum  Inputs=+-
  Constant5 : Constant  Value=pi
  Constant6 : Constant  Value=2*pi
  Constant7 : Constant  Value=pi
  Mod : Math  Operator=mod  SignedPower=on  SaturateOnIntegerOverflow=on
  y : Outport
  wires:
  Constant6/1 -> Mod/2
  Constant5/1 -> Add2/2
  Constant7/1 -> Add3/2
  Mod/1 -> Add3/1  "always_pos"
  Add3/1 -> y/1
  u/1 -> Add2/1
  Add2/1 -> Mod/1

== system dummySpool_cl/dummySpool/Subsystem/non-xcurrent/desiredMoment/Subsystem ==
  u : Inport
  Add2 : Sum  Inputs=+-
  Add3 : Sum  Inputs=+-
  Constant5 : Constant  Value=pi
  Constant6 : Constant  Value=2*pi
  Constant7 : Constant  Value=pi
  Mod : Math  Operator=mod  SignedPower=on  SaturateOnIntegerOverflow=on
  y : Outport
  wires:
  Add3/1 -> y/1
  Add2/1 -> Mod/1
  u/1 -> Add2/1
  Mod/1 -> Add3/1  "always_pos"
  Constant6/1 -> Mod/2
  Constant5/1 -> Add2/2
  Constant7/1 -> Add3/2

== system dummySpool_cl/dummySpool/Subsystem/xcurrent/pathFollowingController/Subsystem2 ==
  posVecGnd : Inport
  gndStnPos : Inport  Port=2
  Atan1 : Trigonometry  Operator=atan2
  Atan2 : Trigonometry  Operator=atan2
  Gain : Gain  Gain=180/pi
  Gain1 : Gain  Gain=180/pi
  Minus : Sum  Inputs=+-
  Selector1 : Selector  InputPortWidth=3  IndexOptions=Index vector (dialog)  Indices=1  OutputSizes=1
  Selector2 : Selector  InputPortWidth=3  IndexOptions=Index vector (dialog)  Indices=[1 2]  OutputSizes=1
  Selector3 : Selector  InputPortWidth=3  IndexOptions=Index vector (dialog)  Indices=3  OutputSizes=1
  Selector4 : Selector  InputPortWidth=3  IndexOptions=Index vector (dialog)  Indices=2  OutputSizes=1
  Sqrt1 : Sqrt  SaturateOnIntegerOverflow=on
  Sqrt2 : Sqrt  SaturateOnIntegerOverflow=on
  Square1 : Math  Operator=square  SignedPower=on  SaturateOnIntegerOverflow=on
  Square2 : Math  Operator=square  SignedPower=on  SaturateOnIntegerOverflow=on
  Sum of Elements : Sum  Inputs=+
  Sum of Elements1 : Sum  Inputs=+
  elevationAngle : Outport
  azimuth Angle : Outport  Port=2
  wires:
  Minus/1 -> Selector4/1, Selector3/1, Selector2/1, Selector1/1
  gndStnPos/1 -> Minus/2
  posVecGnd/1 -> Minus/1
  Sqrt1/1 -> Atan1/2
  Square1/1 -> Sum of Elements/1
  Selector3/1 -> Atan1/1
  Sum of Elements/1 -> Sqrt1/1
  Atan1/1 -> Gain/1
  Selector2/1 -> Square1/1
  Gain/1 -> elevationAngle/1  "elevationAngle"
  Atan2/1 -> Gain1/1
  Square2/1 -> Sum of Elements1/1
  Sum of Elements1/1 -> Sqrt2/1
  Selector1/1 -> Square2/1
  Sqrt2/1 -> Atan2/2
  Selector4/1 -> Atan2/1
  Gain1/1 -> azimuth Angle/1  "azimuthAngle"

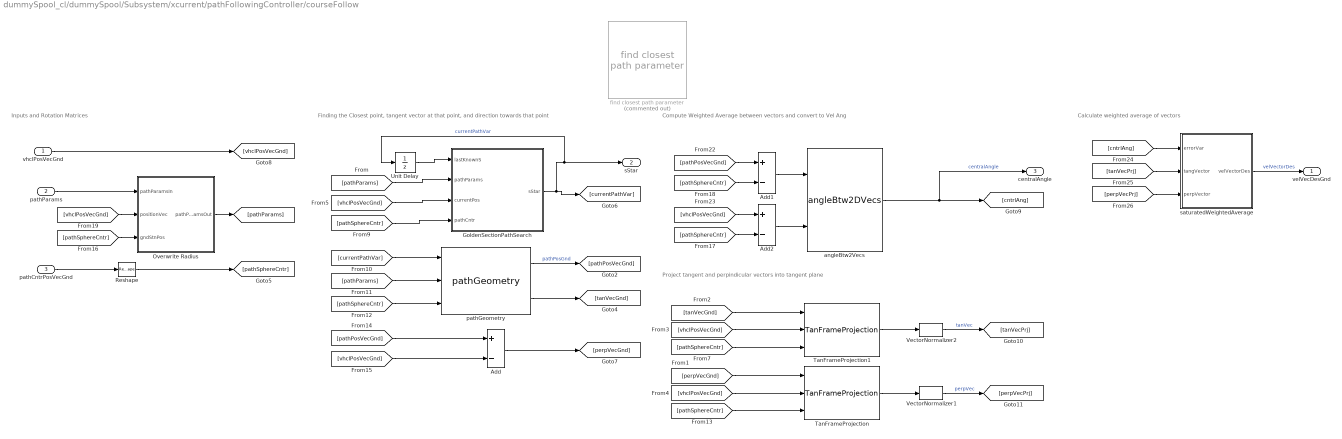
== system dummySpool_cl/dummySpool/Subsystem/xcurrent/pathFollowingController/courseFollow ==
  note: Finding the Closest point, tangent vector at that point, and direction towards that point
  note: Inputs and Rotation Matrices
  note: Compute Weighted Average between vectors and convert to Vel Ang
  note: Project tangent and perpindicular vectors into tangent plane
  note: Calculate weighted average of vectors
  "vhclPosVecGnd " : Inport
  pathParams : Inport  Port=2
  pathCntrPosVecGnd : Inport  Port=3
  Add : Sum  Inputs=+-
  Add1 : Sum  Inputs=+-
  Add2 : Sum  Inputs=+-
  GoldenSectionPathSearch : Subsystem  TreatAsAtomicUnit=on
  Overwrite Radius : Subsystem
  Reshape : Reshape  OutputDimensionality=Column vector (2-D)
  TanFrameProjection : tanFrameProjection_ul/TanFrameProjection  SystemSampleTime=-1  Latency=0  AutoFrameSizeCalculation=off
  TanFrameProjection1 : tanFrameProjection_ul/TanFrameProjection  SystemSampleTime=-1  Latency=0  AutoFrameSizeCalculation=off
  Unit Delay : UnitDelay  SampleTime=-1  HasFrameUpgradeWarning=on
  VectorNormalizer1 : vectorNormalizer_ul/VectorNormalizer   SystemSampleTime=-1  Latency=0  AutoFrameSizeCalculation=off
  VectorNormalizer2 : vectorNormalizer_ul/VectorNormalizer   SystemSampleTime=-1  Latency=0  AutoFrameSizeCalculation=off
  angleBtw2Vecs : angleBtw2Vecs_ul/angleBtw2DVecs  SystemSampleTime=-1  Latency=0  AutoFrameSizeCalculation=off
  find closest path parameter : findClosestPointOnPath_new/find closest path parameter  Commented=on  maxBackward=pathCtrl.searchSize.Value/2  maxForward=pathCtrl.searchSize.Value/2  tau=0.618  convergeTol=1e-4  MaxIters=25
  pathGeometry : pathGeometry_ul/pathGeometry  SystemSampleTime=-1  Latency=0  AutoFrameSizeCalculation=off
  saturatedWeightedAverage : Subsystem  mask{error_upper_lim=pathCtrl.perpErrorVal.Value}
      mask prompts: error_upper_lim "Value of Error yielding 100% perpendicular"
  velVecDesGnd : Outport  VectorParamsAs1DForOutWhenUnconnected=off
  sStar : Outport  Port=2  VectorParamsAs1DForOutWhenUnconnected=off
  centralAngle : Outport  Port=3  VectorParamsAs1DForOutWhenUnconnected=off
  wires:
  saturatedWeightedAverage/1("velVectorDes ") -> velVecDesGnd/1  "velVectorDes"
  [perpVecPrj] -> saturatedWeightedAverage/3("perpVector ")
  [tanVecPrj] -> saturatedWeightedAverage/2(tangVector)
  [cntrlAng] -> saturatedWeightedAverage/1("errorVar ")
  [pathSphereCntr] -> TanFrameProjection/3
  [pathSphereCntr] -> TanFrameProjection1/3
  [vhclPosVecGnd] -> TanFrameProjection/2
  [vhclPosVecGnd] -> TanFrameProjection1/2
  [tanVecGnd] -> TanFrameProjection1/1
  [perpVecGnd] -> TanFrameProjection/1
  [vhclPosVecGnd] -> Overwrite Radius/2(positionVec)
  [pathSphereCntr] -> Overwrite Radius/3(gndStnPos)
  Add2/1 -> angleBtw2Vecs/2
  Add1/1 -> angleBtw2Vecs/1
  [pathSphereCntr] -> Add1/2
  [pathSphereCntr] -> Add2/2
  [pathSphereCntr] -> GoldenSectionPathSearch/4(pathCntr)
  [pathSphereCntr] -> pathGeometry/3
  Reshape/1 -> [pathSphereCntr]
  pathCntrPosVecGnd/1 -> Reshape/1
  Overwrite Radius/1(pathParamsOut) -> [pathParams]
  pathParams/1 -> Overwrite Radius/1(pathParamsIn)
  TanFrameProjection/1 -> VectorNormalizer1/1
  pathGeometry/2 -> [tanVecGnd]
  [pathPosVecGnd] -> Add/1
  [vhclPosVecGnd] -> Add/2
  Add/1 -> [perpVecGnd]
  [pathParams] -> GoldenSectionPathSearch/2(pathParams)
  TanFrameProjection1/1 -> VectorNormalizer2/1
  [currentPathVar] -> pathGeometry/1
  [vhclPosVecGnd] -> Add2/1
  angleBtw2Vecs/1 -> centralAngle/1, [cntrlAng]  "centralAngle"
  VectorNormalizer1/1 -> [perpVecPrj]  "perpVec"
  [pathParams] -> pathGeometry/2
  pathGeometry/1 -> [pathPosVecGnd]  "pathPosGnd"
  "vhclPosVecGnd "/1 -> [vhclPosVecGnd]
  [vhclPosVecGnd] -> GoldenSectionPathSearch/3(currentPos)
  VectorNormalizer2/1 -> [tanVecPrj]  "tanVec"
  [pathPosVecGnd] -> Add1/1
  Unit Delay/1 -> GoldenSectionPathSearch/1(lastKnownS)
  GoldenSectionPathSearch/1(sStar) -> Unit Delay/1, sStar/1, [currentPathVar]  "currentPathVar"
